simulink model "altitude_controller"  (R2018b)
settings: Solver=VariableStepAuto  StartTime=0.0  StopTime=10.0  RelTol=1e-3
values from neighbouring files (symbols this model uses):
  s = r .* exp(1i * (theta + theta0))    [feasibility_study2_flight_time.m]
undefined symbols (not defined in the file or in its folder): C, G
settings Model: Creator=Alistair  LastModifiedBy=Alistair

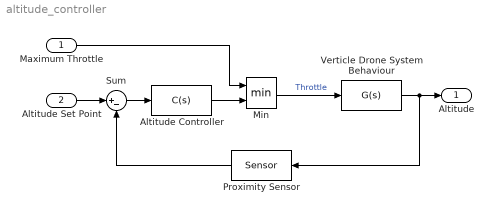
== system altitude_controller ==
  Maximum Throttle : Inport
  Altitude Set Point : Inport  Port=2
  " Proximity Sensor" : Fcn  Expr=Sensor
  Altitude Controller : Fcn  Expr=C(s)
  Min : MinMax  Inputs=2
  Sum : Sum  Inputs=|+-
  "Verticle Drone System Behaviour " : Fcn  Expr=G(s)
  "Altitude " : Outport
  wires:
  "Verticle Drone System Behaviour "/1 -> " Proximity Sensor"/1, "Altitude "/1
  Sum/1 -> Altitude Controller/1
  Altitude Set Point/1 -> Sum/1
  Maximum Throttle/1 -> Min/1
  Altitude Controller/1 -> Min/2
  Min/1 -> "Verticle Drone System Behaviour "/1  "Throttle"
  " Proximity Sensor"/1 -> Sum/2
